simulink subsystem "Piero"  (R2023b)
settings: Solver=VariableStepAuto  StartTime=0.0  StopTime=10.0  RelTol=1e-3
settings Model: Creator=Enrique  LastModifiedBy=Enrique

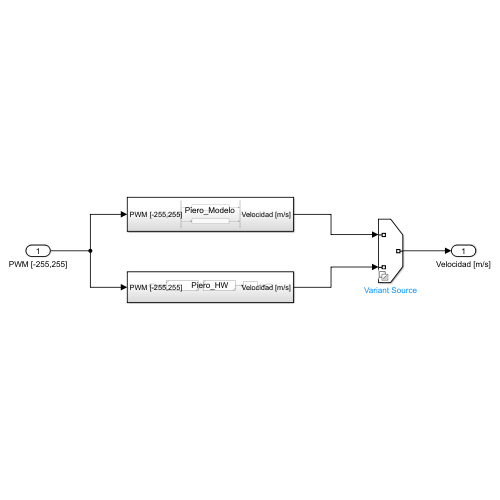
[thumbnail: Simulink's stored preview of the top-level diagram]
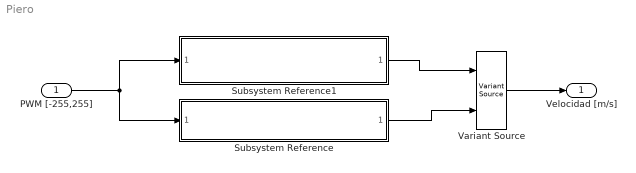
== system Piero ==
  PWM [-255,255] : Inport
  Subsystem Reference : Subsystem  ReferencedSubsystem=Piero_HW
  Subsystem Reference1 : Subsystem  ReferencedSubsystem=Piero_Modelo
  Variant Source : VariantSource  VariantControlMode=sim codegen switching
  Velocidad [m/s] : Outport
  wires:
  PWM [-255,255]/1 -> Subsystem Reference/1, Subsystem Reference1/1
  Variant Source/1 -> Velocidad [m/s]/1
  Subsystem Reference/1 -> Variant Source/2
  Subsystem Reference1/1 -> Variant Source/1
